simulink model "Emmanuel_Mati_Simulink_Project_P_Control"  (R2020a)
settings: Solver=VariableStepAuto  StartTime=0.0  StopTime=10  RelTol=1e-3
settings Model: Creator=mati1  LastModifiedBy=mati1

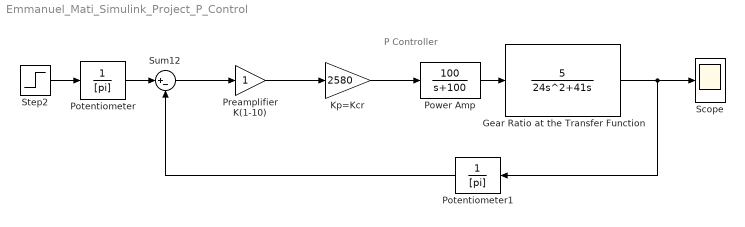
== system Emmanuel_Mati_Simulink_Project_P_Control ==
  note: P Controller
  Gear Ratio at the Transfer Function : TransferFcn  Numerator=[5]  Denominator=[24 41 0]
  Kp=Kcr : Gain  Gain=2580
  Potentiometer : TransferFcn  Denominator=[pi]
  Potentiometer1 : TransferFcn  Denominator=[pi]
  Power Amp : TransferFcn  Numerator=[100]  Denominator=[1 100]
  Preamplifier K(1-10) : Gain
  Scope : Scope
  Step2 : Step  Before=1  SampleTime=0
  Sum12 : Sum  Inputs=|+-
  wires:
  Preamplifier K(1-10)/1 -> Kp=Kcr/1
  Sum12/1 -> Preamplifier K(1-10)/1
  Gear Ratio at the Transfer Function/1 -> Scope/1, Potentiometer1/1
  Power Amp/1 -> Gear Ratio at the Transfer Function/1
  Potentiometer/1 -> Sum12/1
  Potentiometer1/1 -> Sum12/2
  Step2/1 -> Potentiometer/1
  Kp=Kcr/1 -> Power Amp/1
